simulink model "b_2x_8a_r309a"  (Simulink 6.2)
settings: Solver=ode45  StartTime=0.0  StopTime=1030.0  RelTol=1e-3
undefined symbols (not defined in the file): ant_bits, BEE2_usr, blockCountBits, blockRowBits, cmult_4bit_em
libraries: xbsIndex_r3 x3300, xps_library x102, casper_library x96
(part 8 of 22)

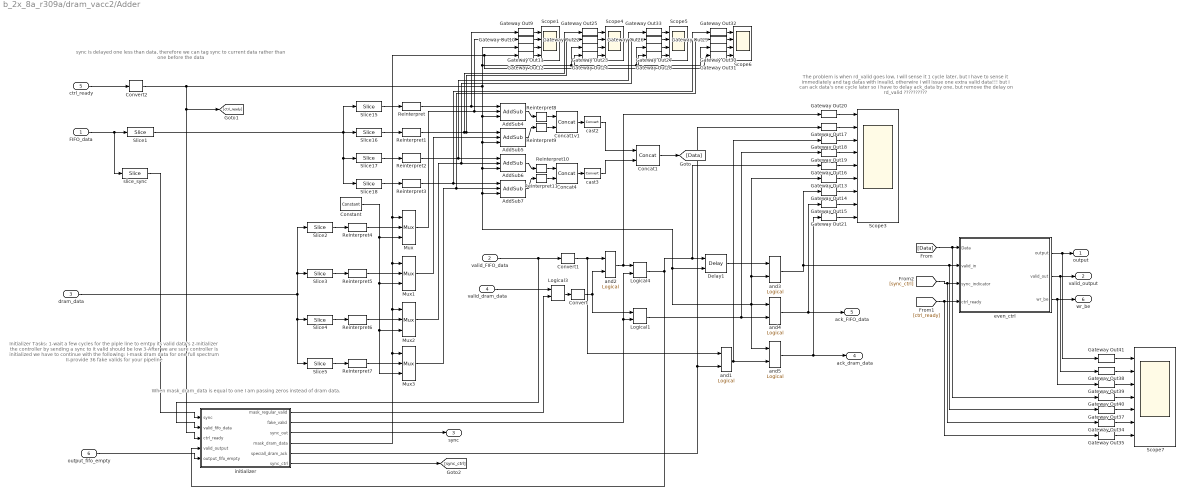
== system b_2x_8a_r309a/dram_vacc2/Adder ==
  note: When mask_dram_data is equal to one
      | I am passing zeros instead of dram data.
  note: Initializer Tasks:
      | 1-wait a few cycles for the piple line to emtpy
      | its valid data's
      | 2-Initializer the controller by sending a sync to it
      | valid should be low
      | 3-After we are sure controller is initialized we have to
      | continue with the following:
      | I-mask dram data for one full spectrum
      | II-provide 36 fake valids for your pipeline
  note: The problem is when rd_valid goes low, I will sense it 1 cycle later,
      | but I have to sense it immediately and tag datas with invalid,
      | otherwire I will issue one extra valid data!!!
      | but I can ack data's one cycle later so
      | I have to delay ack_data by one, but remove the delay on rd_valid
      | ??????????
  note: sync is delayed one less than data,
      | therefore we can tag sync to current data rather than
      | one before the data
  FIFO_data : Inport  Port=1  LatchInput=off
  valid_FIFO_data : Inport  Port=2  LatchInput=off
  dram_data : Inport  Port=3  LatchInput=off
  valid_dram_data : Inport  Port=4  LatchInput=off
  ctrl_ready : Inport  Port=5  LatchInput=off
  output_fifo_empty : Inport  Port=6  LatchInput=off
  AddSub{4..7} (4 alike) : xbsIndex_r3/AddSub  mode=Addition  precision=User Defined  arith_type="Signed  (2's comp)"  n_bits=32  bin_pt=0  quantization="Round  (unbiased: +/- Inf)"  overflow=Wrap  latency=3  explicit_period=on  period=1  use_carryin=off  use_carryout=off  en=on  dbl_ovrd=off  show_param=off  use_core=on  pipeline=on  use_rpm=on  gen_core=off
      settings: xl_area=[0, 0, 0, 0, 0, 0, 0]
  Concat1 : xbsIndex_r3/Concat  num_inputs=2  explicit_period=off  period=1  dbl_ovrd=off
  Concat1v1 : xbsIndex_r3/Concat  num_inputs=2  explicit_period=off  period=1  dbl_ovrd=off
  Concat4 : xbsIndex_r3/Concat  num_inputs=2  explicit_period=off  period=1  dbl_ovrd=off
  Constant : xbsIndex_r3/Constant  const=0  equ=P=C  arith_type="Signed  (2's comp)"  n_bits=32  bin_pt=0  opselect=C  inp2=PCIN>>17  opr=+  inp1=P  carry=CIN  iostate=0  explicit_period=on  period=1  dbl_ovrd=off
  Convert : xbsIndex_r3/Convert  arith_type=Boolean  n_bits=8  bin_pt=6  quantization=Truncate  overflow=Wrap  latency=0  explicit_period=off  period=1  dbl_ovrd=off  show_param=off  inserted_by_tool=off  pipeline=off
      settings: xl_area=[0, 0, 0, 0, 0, 0, 0]
  Convert1 : xbsIndex_r3/Convert  arith_type=Boolean  n_bits=8  bin_pt=6  quantization=Truncate  overflow=Wrap  latency=0  explicit_period=off  period=1  dbl_ovrd=off  show_param=off  inserted_by_tool=off  pipeline=off
      settings: xl_area=[0, 0, 0, 0, 0, 0, 0]
  Convert2 : xbsIndex_r3/Convert  arith_type=Boolean  n_bits=8  bin_pt=6  quantization=Truncate  overflow=Wrap  latency=0  explicit_period=off  period=1  dbl_ovrd=off  show_param=off  inserted_by_tool=off  pipeline=off
      settings: xl_area=[0, 0, 0, 0, 0, 0, 0]
  Delay1 : xbsIndex_r3/Delay  latency=3  reg_retiming=off  explicit_period=on  period=1  en=on  accept_only_valid=off  init_zero=on  dbl_ovrd=off  show_param=off
      settings: xl_area=[0, 0, 0, 0, 0, 0, 0]
  Gateway Out{9..35,37..41} (32 alike) : xbsIndex_r3/Gateway Out  output_type=Double  nbits=8  bin_pt=6  arith_type=Boolean  quantization=Truncate  overflow=Wrap  hdl_port=off  timing_constraint=None  locs_specified=off  LOCs={}  needs_fixed_name=off  show_param=off
      settings: xl_area=[0, 0, 0, 0, 0, 0, 0]
  Logical1 : xbsIndex_r3/Logical  logical_function=OR  inputs=2  precision=Full  arith_type=Unsigned  n_bits=8  bin_pt=2  align_bp=on  latency=0  explicit_period=off  period=1  en=off  dbl_ovrd=off  show_param=off
      settings: xl_area=[0, 0, 0, 0, 0, 0, 0]
  Logical3 : xbsIndex_r3/Logical  logical_function=AND  inputs=2  precision=Full  arith_type=Unsigned  n_bits=8  bin_pt=2  align_bp=on  latency=0  explicit_period=off  period=1  en=off  dbl_ovrd=off  show_param=off
      settings: xl_area=[0, 0, 0, 0, 0, 0, 0]
  Logical4 : xbsIndex_r3/Logical  logical_function=OR  inputs=2  precision=Full  arith_type=Unsigned  n_bits=8  bin_pt=2  align_bp=on  latency=0  explicit_period=off  period=1  en=off  dbl_ovrd=off  show_param=off
      settings: xl_area=[0, 0, 0, 0, 0, 0, 0]
  Mux{,1..3} (4 alike) : xbsIndex_r3/Mux  inputs=2  precision=Full  arith_type="Signed  (2's comp)"  n_bits=8  bin_pt=2  quantization=Truncate  overflow=Wrap  latency=0  explicit_period=off  period=1  en=off  dbl_ovrd=off  show_param=off  mux_type=off  use_rpm=off  gen_core=off
      settings: xl_area=[0, 0, 0, 0, 0, 0, 0]
  Reinterpret{,1..7} (8 alike) : xbsIndex_r3/Reinterpret  force_arith_type=on  arith_type="Signed  (2's comp)"  force_bin_pt=on  bin_pt=0  force_valid=on
  Reinterpret{8..11} (4 alike) : xbsIndex_r3/Reinterpret  force_arith_type=on  arith_type=Unsigned  force_bin_pt=on  bin_pt=0  force_valid=on
  Scope{1,4..6} (4 alike) : Scope  NumInputPorts=4
      Scope1 settings: YMin=0~0~0~-1  YMax=1~1750~1~1  SaveName=ScopeData30
      Scope4 settings: YMin=0~0~0~-1  YMax=1~1750~1~1  SaveName=ScopeData4
      Scope5 settings: YMin=0~0~0~-1  YMax=1~1750~1~1  SaveName=ScopeData5
      Scope6 settings: YMin=0~0~0~-1  YMax=1~1750~1~1  SaveName=ScopeData6
  Scope3 : Scope  NumInputPorts=9
      settings: YMin=0~0~0~-1~-5~-5~-5~-5~-5  YMax=1~1750~1~1~5~5~5~5~5  SaveName=ScopeData11
  Scope7 : Scope  NumInputPorts=7
      settings: YMin=0~0~0~-1~-5~-5~-5  YMax=1~1750~1~1~5~5~5  SaveName=ScopeData36
  Slice1 : xbsIndex_r3/Slice  mode=Lower Bit Location + Width  nbits=128  bit1=0  base1=MSB of Input  bit0=0  base0=LSB of Input  boolean_output=off  explicit_period=off  period=1  dbl_ovrd=off
  Slice15 : xbsIndex_r3/Slice  mode=Lower Bit Location + Width  nbits=32  bit1=96  base1=MSB of Input  bit0=96  base0=LSB of Input  boolean_output=off  explicit_period=off  period=1  dbl_ovrd=off
  Slice16 : xbsIndex_r3/Slice  mode=Lower Bit Location + Width  nbits=32  bit1=-32  base1=MSB of Input  bit0=64  base0=LSB of Input  boolean_output=off  explicit_period=off  period=1  dbl_ovrd=off
  Slice17 : xbsIndex_r3/Slice  mode=Lower Bit Location + Width  nbits=32  bit1=0  base1=MSB of Input  bit0=32  base0=LSB of Input  boolean_output=off  explicit_period=off  period=1  dbl_ovrd=off
  Slice18 : xbsIndex_r3/Slice  mode=Lower Bit Location + Width  nbits=32  bit1=0  base1=MSB of Input  bit0=0  base0=LSB of Input  boolean_output=off  explicit_period=off  period=1  dbl_ovrd=off
  Slice2 : xbsIndex_r3/Slice  mode=Lower Bit Location + Width  nbits=32  bit1=0  base1=MSB of Input  bit0=104  base0=LSB of Input  boolean_output=off  explicit_period=off  period=1  dbl_ovrd=off
  Slice3 : xbsIndex_r3/Slice  mode=Lower Bit Location + Width  nbits=32  bit1=72  base1=MSB of Input  bit0=72  base0=LSB of Input  boolean_output=off  explicit_period=off  period=1  dbl_ovrd=off
  Slice4 : xbsIndex_r3/Slice  mode=Lower Bit Location + Width  nbits=32  bit1=0  base1=MSB of Input  bit0=32  base0=LSB of Input  boolean_output=off  explicit_period=off  period=1  dbl_ovrd=off
  Slice5 : xbsIndex_r3/Slice  mode=Lower Bit Location + Width  nbits=32  bit1=0  base1=MSB of Input  bit0=0  base0=LSB of Input  boolean_output=off  explicit_period=off  period=1  dbl_ovrd=off
  and1 : xbsIndex_r3/Logical  logical_function=OR  inputs=2  precision=Full  arith_type=Unsigned  n_bits=8  bin_pt=2  align_bp=on  latency=0  explicit_period=off  period=1  en=off  dbl_ovrd=off  show_param=off
      settings: xl_area=[0, 0, 0, 0, 0, 0, 0]
  and{2..5} (4 alike) : xbsIndex_r3/Logical  logical_function=AND  inputs=2  precision=Full  arith_type=Unsigned  n_bits=8  bin_pt=2  align_bp=on  latency=0  explicit_period=off  period=1  en=off  dbl_ovrd=off  show_param=off
      settings: xl_area=[0, 0, 0, 0, 0, 0, 0]
  cast2 : xbsIndex_r3/Convert  arith_type=Unsigned  n_bits=72  bin_pt=0  quantization=Truncate  overflow=Wrap  latency=0  explicit_period=off  period=1  dbl_ovrd=off  show_param=off  inserted_by_tool=off  pipeline=off
      settings: xl_area=[0, 0, 0, 0, 0, 0, 0]
  cast3 : xbsIndex_r3/Convert  arith_type=Unsigned  n_bits=72  bin_pt=0  quantization=Truncate  overflow=Wrap  latency=0  explicit_period=off  period=1  dbl_ovrd=off  show_param=off  inserted_by_tool=off  pipeline=off
      settings: xl_area=[0, 0, 0, 0, 0, 0, 0]
  even_ctrl : Subsystem
  initializer : Subsystem
  slice_sync : xbsIndex_r3/Slice  mode=Upper Bit Location + Width  nbits=1  bit1=0  base1=MSB of Input  bit0=0  base0=LSB of Input  boolean_output=on  explicit_period=off  period=1  dbl_ovrd=off
  output : Outport
  valid_output : Outport  Port=2
  sync : Outport  Port=3
  ack_dram_data : Outport  Port=4
  ack_FIFO_data : Outport  Port=5
  wr_be : Outport  Port=6
  wires:
  Gateway Out31/1 -> Scope6/4
  Gateway Out30/1 -> Scope6/3
  Gateway Out29/1 -> Scope6/2
  Gateway Out32/1 -> Scope6/1
  Gateway Out28/1 -> Scope5/4
  Gateway Out27/1 -> Scope5/3
  Gateway Out26/1 -> Scope5/2
  Gateway Out33/1 -> Scope5/1
  Gateway Out24/1 -> Scope4/4
  Gateway Out23/1 -> Scope4/3
  Gateway Out22/1 -> Scope4/2
  Gateway Out25/1 -> Scope4/1
  Reinterpret11/1 -> Concat4/2
  Reinterpret10/1 -> Concat4/1
  Reinterpret9/1 -> Concat1v1/2
  Reinterpret8/1 -> Concat1v1/1
  Reinterpret7/1 -> Mux3/2
  Reinterpret6/1 -> Mux2/2
  Reinterpret5/1 -> Mux1/2
  Reinterpret4/1 -> Mux/2
  Reinterpret3/1 -> Gateway Out32/1, AddSub7/1
  Reinterpret2/1 -> Gateway Out33/1, AddSub6/1
  Reinterpret1/1 -> Gateway Out22/1, AddSub5/1, Gateway Out25/1
  Reinterpret/1 -> Gateway Out9/1, AddSub4/1
  Logical1/1 -> Gateway Out19/1, and4/2
  Gateway Out21/1 -> Scope3/9
  Gateway Out15/1 -> Scope3/8
  Gateway Out14/1 -> Scope3/7
  Gateway Out13/1 -> Scope3/6
  Gateway Out16/1 -> Scope3/5
  Gateway Out18/1 -> Scope3/3
  Gateway Out19/1 -> Scope3/4
  Gateway Out17/1 -> Scope3/2
  Gateway Out20/1 -> Scope3/1
  and1/1 -> Gateway Out18/1, and5/2
  and5/1 -> Gateway Out21/1, ack_dram_data/1
  Logical4/1 -> Gateway Out16/1, Delay1/1, initializer/4(valid_output)
  Gateway Out12/1 -> Scope1/4
  Gateway Out11/1 -> Scope1/3
  Gateway Out10/1 -> Scope1/2
  Gateway Out9/1 -> Scope1/1
  initializer/5(speciall_dram_ack) -> Gateway Out17/1, and1/2
  output_fifo_empty/1 -> initializer/5(output_fifo_empty)
  Constant/1 -> Mux2/3, Mux3/3, Mux1/3, Mux/3
  initializer/4(mask_dram_data) -> Mux3/1, Mux2/1, Gateway Out31/1, Gateway Out28/1, Gateway Out24/1, Gateway Out12/1, Mux/1, Mux1/1
  Slice2/1 -> Reinterpret4/1
  Slice3/1 -> Reinterpret5/1
  Slice4/1 -> Reinterpret6/1
  Slice5/1 -> Reinterpret7/1
  initializer/3(sync_out) -> sync/1
  and2/1 -> Gateway Out20/1, Logical4/1
  and4/1 -> Gateway Out15/1, ack_FIFO_data/1
  Delay1/1 -> and3/1
  initializer/2(fake_valid) -> Logical1/2, Logical4/2
  Logical3/1 -> Convert/1
  initializer/1(mask_regular_valid) -> Logical3/2
  valid_dram_data/1 -> Logical3/1
  and3/1 -> Gateway Out14/1, even_ctrl/2(valid_in), Gateway Out37/1
  Convert2/1 -> Gateway Out30/1, Gateway Out27/1, Gateway Out23/1, Gateway Out11/1, AddSub4/3, AddSub5/3, Delay1/2, Gateway Out13/1, and3/2, and5/1, and4/1, AddSub7/3, AddSub6/3, [ctrl_ready], initializer/3(ctrl_ready)
  Convert1/1 -> and1/1, and2/1
  Convert/1 -> Logical1/1, and2/2
  slice_sync/1 -> initializer/1(sync)
  Slice1/1 -> Slice18/1, Slice17/1, Slice16/1, Slice15/1
  dram_data/1 -> Slice4/1, Slice5/1, Slice3/1, Slice2/1
  valid_FIFO_data/1 -> Convert1/1, initializer/2(valid_fifo_data)
  ctrl_ready/1 -> Convert2/1
  FIFO_data/1 -> slice_sync/1, Slice1/1
  cast3/1 -> Concat1/2
  Concat4/1 -> cast3/1
  cast2/1 -> Concat1/1
  Concat1v1/1 -> cast2/1
  AddSub7/1 -> Reinterpret11/1
  AddSub6/1 -> Reinterpret10/1
  AddSub5/1 -> Reinterpret9/1
  AddSub4/1 -> Reinterpret8/1
  Mux3/1 -> Gateway Out29/1, AddSub7/2
  Mux2/1 -> Gateway Out26/1, AddSub6/2
  Mux1/1 -> AddSub5/2
  Mux/1 -> Gateway Out10/1, AddSub4/2
  Slice18/1 -> Reinterpret3/1
  Slice17/1 -> Reinterpret2/1
  Slice16/1 -> Reinterpret1/1
  Slice15/1 -> Reinterpret/1
  even_ctrl/1(output) -> output/1, Gateway Out41/1
  even_ctrl/2(valid_out) -> valid_output/1, Gateway Out38/1
  Concat1/1 -> [Data]
  [Data] -> even_ctrl/1(Data), Gateway Out40/1
  [ctrl_ready] -> even_ctrl/4(ctrl_ready), Gateway Out35/1
  even_ctrl/3(wr_be) -> wr_be/1, Gateway Out39/1
  initializer/6(sync_ctrl) -> [sync_ctrl]
  [sync_ctrl] -> even_ctrl/3(sync_indicator), Gateway Out34/1
  Gateway Out35/1 -> Scope7/7
  Gateway Out34/1 -> Scope7/6
  Gateway Out37/1 -> Scope7/5
  Gateway Out39/1 -> Scope7/3
  Gateway Out40/1 -> Scope7/4
  Gateway Out38/1 -> Scope7/2
  Gateway Out41/1 -> Scope7/1

== system b_2x_8a_r309a/dram_vacc2/RB_reg ==
  note: HIgh bit of tag means its a read back
      | and low bit means its a valid read back
      | This module has to ack dram for all
      | rd backs (even invalid ones)
      | but it neads to only capture valid
      | read backs.
  note: if this is high it means data is a RB data
  dram_data : Inport  Port=1  LatchInput=off
  rd_tag : Inport  Port=2  LatchInput=off
  rd_valid : Inport  Port=3  LatchInput=off
  dram_rd_ack : Inport  Port=4  LatchInput=off
  ack_RB : Inport  Port=5  LatchInput=off
  RB_active : Inport  Port=6  LatchInput=off
  Concat : xbsIndex_r3/Concat  num_inputs=2  explicit_period=off  period=1  dbl_ovrd=off
  Convert{1..2,4..5} (4 alike) : xbsIndex_r3/Convert  arith_type=Boolean  n_bits=31  bin_pt=0  quantization=Truncate  overflow=Wrap  latency=0  explicit_period=off  period=1  dbl_ovrd=off  show_param=off  inserted_by_tool=off  pipeline=off
      settings: xl_area=[0, 0, 0, 0, 0, 0, 0]
  Delay : xbsIndex_r3/Delay  latency=1  reg_retiming=on  explicit_period=off  period=1  en=off  accept_only_valid=off  init_zero=on  dbl_ovrd=off  show_param=off
      settings: xl_area=[0, 0, 0, 0, 0, 0, 0]
  Inverter2 : xbsIndex_r3/Inverter  latency=0  explicit_period=off  period=1  en=off  dbl_ovrd=off  show_param=off
      settings: xl_area=[0, 0, 0, 0, 0, 0, 0]
  Logical1 : xbsIndex_r3/Logical  logical_function=AND  inputs=2  precision=Full  arith_type=Unsigned  n_bits=8  bin_pt=2  align_bp=on  latency=0  explicit_period=on  period=1  en=off  dbl_ovrd=off  show_param=off
      settings: xl_area=[0, 0, 0, 0, 0, 0, 0]
  Logical2 : xbsIndex_r3/Logical  logical_function=AND  inputs=4  precision=Full  arith_type=Unsigned  n_bits=8  bin_pt=2  align_bp=on  latency=0  explicit_period=on  period=1  en=off  dbl_ovrd=off  show_param=off
      settings: xl_area=[0, 0, 0, 0, 0, 0, 0]
  Logical3 : xbsIndex_r3/Logical  logical_function=AND  inputs=2  precision=Full  arith_type=Unsigned  n_bits=8  bin_pt=2  align_bp=on  latency=0  explicit_period=on  period=1  en=off  dbl_ovrd=off  show_param=off
      settings: xl_area=[0, 0, 0, 0, 0, 0, 0]
  Logical4 : xbsIndex_r3/Logical  logical_function=OR  inputs=2  precision=Full  arith_type=Unsigned  n_bits=8  bin_pt=2  align_bp=on  latency=0  explicit_period=on  period=1  en=off  dbl_ovrd=off  show_param=off
      settings: xl_area=[0, 0, 0, 0, 0, 0, 0]
  Register : xbsIndex_r3/Register  init=0  reg_only_valid=off  explicit_period=off  period=1  rst=on  en=on  out_en=off  dbl_ovrd=off  show_param=off
      settings: xl_area=[0, 0, 0, 0, 0, 0, 0]
  Reinterpret : xbsIndex_r3/Reinterpret  force_arith_type=on  arith_type=Unsigned  force_bin_pt=on  bin_pt=0  force_valid=on
  Slice : xbsIndex_r3/Slice  mode=Lower Bit Location + Width  nbits=64  bit1=0  base1=MSB of Input  bit0=72  base0=LSB of Input  boolean_output=off  explicit_period=off  period=1  dbl_ovrd=off
  Slice1 : xbsIndex_r3/Slice  mode=Lower Bit Location + Width  nbits=64  bit1=0  base1=MSB of Input  bit0=0  base0=LSB of Input  boolean_output=off  explicit_period=off  period=1  dbl_ovrd=off
  Slice2 : xbsIndex_r3/Slice  mode=Upper Bit Location + Width  nbits=1  bit1=0  base1=MSB of Input  bit0=74  base0=LSB of Input  boolean_output=on  explicit_period=off  period=1  dbl_ovrd=off
  Slice3 : xbsIndex_r3/Slice  mode=Lower Bit Location + Width  nbits=1  bit1=0  base1=MSB of Input  bit0=0  base0=LSB of Input  boolean_output=on  explicit_period=off  period=1  dbl_ovrd=off
  Trickle_FWFT : Subsystem  mask{depth=16}
      mask init:
      | cursys = gcb ; 
      | set_param([cursys, '/FIFO'], 'depth', depth);
      mask StyleString: popup(16|32|64|128|256|512|1K|2K|4K|8K|16K|32K|64K)
  posedge : Subsystem
  dout : Outport
  valid : Outport  Port=2
  ack_dram : Outport  Port=3
  en_addr_gen : Outport  Port=4
  wires:
  Reinterpret/1 -> Inverter2/1
  Convert2/1 -> Logical3/1
  Slice3/1 -> Logical2/4
  Slice2/1 -> Logical1/1
  Convert4/1 -> Logical1/2
  Logical4/1 -> Register/2
  Register/1 -> Logical3/2
  Logical3/1 -> Logical4/2, en_addr_gen/1
  Inverter2/1 -> Convert2/1
  Trickle_FWFT/4(%full) -> Reinterpret/1
  Trickle_FWFT/2(valid) -> valid/1
  Trickle_FWFT/1(data_out) -> dout/1
  posedge/1(out) -> Logical4/1, Trickle_FWFT/4(reset)
  Concat/1 -> Trickle_FWFT/1(din)
  ack_RB/1 -> Trickle_FWFT/3(ack)
  Convert1/1 -> Logical2/3, posedge/1(in)
  dram_data/1 -> Slice1/1, Slice/1
  Slice1/1 -> Concat/2
  Slice/1 -> Concat/1
  Convert5/1 -> Logical2/2
  RB_active/1 -> Convert1/1
  Logical2/1 -> Register/3, Register/1, Trickle_FWFT/2(we)
  dram_rd_ack/1 -> Convert5/1
  Logical1/1 -> Logical2/1, Delay/1
  Delay/1 -> ack_dram/1
  rd_valid/1 -> Convert4/1
  rd_tag/1 -> Slice3/1, Slice2/1

== system b_2x_8a_r309a/dram_vacc2/Trickle_FWFT ==
  note: We needed a FIFO which brings the valid data automatically to the output.
      | The regular XILINX Fifos are not FWFT (First Word Fall Through).
      | We tried to make one but it was really hard to make one agreeing with the exact specs.
      | This module which we have named it Trickle_FWFT Fifo works very similiarly with minor
      | differences which servers our purpose here in the DRAM VACC module.
  note: The real depth of this module is depth+1.
      | The valid signal will go high with one cycle delay.
  din : Inport  Port=1  LatchInput=off
  we : Inport  Port=2  LatchInput=off
  ack : Inport  Port=3  LatchInput=off
  reset : Inport  Port=4  LatchInput=off
  Convert : xbsIndex_r3/Convert  Orientation=left  arith_type=Boolean  n_bits=8  bin_pt=6  quantization=Truncate  overflow=Wrap  latency=0  explicit_period=on  period=1  dbl_ovrd=off  show_param=off  inserted_by_tool=off  pipeline=off
      settings: xl_area=[0, 0, 0, 0, 0, 0, 0]
  Convert1 : xbsIndex_r3/Convert  arith_type=Boolean  n_bits=8  bin_pt=6  quantization=Truncate  overflow=Wrap  latency=0  explicit_period=off  period=1  dbl_ovrd=off  show_param=off  inserted_by_tool=off  pipeline=off
      settings: xl_area=[0, 0, 0, 0, 0, 0, 0]
  Convert2 : xbsIndex_r3/Convert  arith_type=Boolean  n_bits=8  bin_pt=6  quantization=Truncate  overflow=Wrap  latency=0  explicit_period=off  period=1  dbl_ovrd=off  show_param=off  inserted_by_tool=off  pipeline=off
      settings: xl_area=[0, 0, 0, 0, 0, 0, 0]
  FIFO : xbsIndex_r3/FIFO  depth=512  percent_nbits=1  store_only_valid=on  init_zero=on  explicit_period=on  period=1  rst=on  en=off  use_almost_empty=off  almost_empty_offset=6  use_almost_full=off  almost_full_offset=6  dbl_ovrd=off  show_param=off  mem_type=Block RAM  gen_core=off
      settings: xl_area=[0, 0, 0, 0, 0, 0, 0]
  Inverter3 : xbsIndex_r3/Inverter  latency=0  explicit_period=off  period=1  en=off  dbl_ovrd=off  show_param=off
      settings: xl_area=[0, 0, 0, 0, 0, 0, 0]
  Logical2 : xbsIndex_r3/Logical  logical_function=OR  inputs=2  precision=Full  arith_type=Unsigned  n_bits=8  bin_pt=2  align_bp=on  latency=0  explicit_period=on  period=1  en=off  dbl_ovrd=off  show_param=off
      settings: xl_area=[0, 0, 0, 0, 0, 0, 0]
  not_valid : xbsIndex_r3/Register  init=1  reg_only_valid=off  explicit_period=on  period=1  rst=on  en=on  out_en=off  dbl_ovrd=off  show_param=off
      settings: xl_area=[0, 0, 0, 0, 0, 0, 0]
  data_out : Outport
  valid : Outport  Port=2
  full : Outport  Port=3
  %full : Outport  Port=4
  wires:
  din/1 -> FIFO/1
  we/1 -> FIFO/2
  FIFO/2 -> not_valid/1
  ack/1 -> Convert2/1
  FIFO/1 -> data_out/1
  FIFO/4 -> full/1
  Inverter3/1 -> valid/1
  reset/1 -> FIFO/4, not_valid/2
  Logical2/1 -> FIFO/3, not_valid/3
  not_valid/1 -> Convert1/1
  Convert/1 -> Logical2/1
  FIFO/3 -> %full/1
  Convert1/1 -> Inverter3/1, Convert/1
  Convert2/1 -> Logical2/2

== system b_2x_8a_r309a/dram_vacc2/ctrl_unit ==
  valid_data : Inport  Port=1  LatchInput=off
  sync : Inport  Port=2  LatchInput=off
  en_RB_addr : Inport  Port=3  LatchInput=off
  Concat1 : xbsIndex_r3/Concat  num_inputs=3  explicit_period=off  period=1  dbl_ovrd=off
  Convert2 : xbsIndex_r3/Convert  arith_type=Unsigned  n_bits=30  bin_pt=0  quantization=Truncate  overflow=Wrap  latency=0  explicit_period=off  period=1  dbl_ovrd=off  show_param=off  inserted_by_tool=off  pipeline=off
      settings: xl_area=[0, 0, 0, 0, 0, 0, 0]
  Delay1 : xbsIndex_r3/Delay  latency=2  reg_retiming=off  explicit_period=on  period=1  en=off  accept_only_valid=off  init_zero=on  dbl_ovrd=off  show_param=off
      settings: xl_area=[0, 0, 0, 0, 0, 0, 0]
  Delay2 : xbsIndex_r3/Delay  latency=1  reg_retiming=off  explicit_period=on  period=1  en=off  accept_only_valid=off  init_zero=on  dbl_ovrd=off  show_param=off
      settings: xl_area=[0, 0, 0, 0, 0, 0, 0]
  Mux : xbsIndex_r3/Mux  inputs=2  precision=Full  arith_type="Signed  (2's comp)"  n_bits=8  bin_pt=2  quantization=Truncate  overflow=Wrap  latency=0  explicit_period=off  period=1  en=off  dbl_ovrd=off  show_param=off  mux_type=off  use_rpm=off  gen_core=off
      settings: xl_area=[0, 0, 0, 0, 0, 0, 0]
  Mux2 : xbsIndex_r3/Mux  inputs=2  precision=Full  arith_type="Signed  (2's comp)"  n_bits=8  bin_pt=2  quantization=Truncate  overflow=Wrap  latency=0  explicit_period=off  period=1  en=off  dbl_ovrd=off  show_param=off  mux_type=off  use_rpm=off  gen_core=off
      settings: xl_area=[0, 0, 0, 0, 0, 0, 0]
  RB_active_or_finish : Subsystem
  address_gen_vacc_DRAM : Subsystem  mask{acc_length=acc_length, valid_length=burst_length}
      mask prompts: acc_length "Accumulation length?"; valid_length "Valid period length?"
      mask init:
      | address_gen_vacc_v2_mask;
  cmd_gen : Subsystem
  latch_rb_enable : Subsystem
  negedge : Subsystem  Orientation=down
  readback_address_dram_vacc : Subsystem  mask{acc_length=acc_length, valid_length=valid_length}
      mask prompts: acc_length "Accumulation length?"; valid_length "Valid period length?"
      mask init:
      | readback_address_dram_vacc_mask;
  address : Outport
  cmd_tag : Outport  Port=2
  RB_active : Outport  Port=3
  RWn : Outport  Port=4
  cmd_valid : Outport  Port=5
  ready : Outport  Port=6
  wires:
  latch_rb_enable/2(cmd_tag) -> Concat1/3
  Delay1/1 -> latch_rb_enable/1(sync), readback_address_dram_vacc/1(sync)  "v"
  negedge/1(out) -> latch_rb_enable/3(negedge)
  latch_rb_enable/1(inc_addr_en) -> RB_active_or_finish/1(enable_rb_addr), readback_address_dram_vacc/2(en)
  readback_address_dram_vacc/1(readback_addr) -> Mux2/3
  valid_data/1 -> cmd_gen/1(valid_data)
  cmd_gen/6(rb_addr_en) -> negedge/1(in), Concat1/1, Mux2/1
  cmd_gen/5(ready) -> ready/1
  cmd_gen/4(cmd_valid) -> cmd_valid/1
  cmd_gen/3(RWn) -> Mux/1, RWn/1
  RB_active_or_finish/1(rb_active) -> RB_active/1
  Mux2/1 -> address/1, Convert2/1
  en_RB_addr/1 -> latch_rb_enable/2(rb_addr_enable)
  Delay2/1 -> address_gen_vacc_DRAM/1(sync)
  Concat1/1 -> cmd_tag/1
  Convert2/1 -> Concat1/2
  cmd_gen/2(wr_addr_en) -> address_gen_vacc_DRAM/3(write_en)
  cmd_gen/1(re_addr_en) -> address_gen_vacc_DRAM/2(read_en)
  Mux/1 -> Mux2/2
  address_gen_vacc_DRAM/2(read_addr) -> Mux/3
  address_gen_vacc_DRAM/1(write_addr) -> Mux/2
  sync/1 -> Delay2/1, RB_active_or_finish/2(sync), Delay1/1, cmd_gen/2(sync)

== system b_2x_8a_r309a/dram_vacc2/dram1 ==
  rst : Inport  Port=1  LatchInput=off
  address : Inport  Port=2  LatchInput=off
  data_in : Inport  Port=3  LatchInput=off
  wr_be : Inport  Port=4  LatchInput=off
  RWn : Inport  Port=5  LatchInput=off
  cmd_tag : Inport  Port=6  LatchInput=off
  cmd_valid : Inport  Port=7  LatchInput=off
  rd_ack : Inport  Port=8  LatchInput=off
  Constant : Constant  Value=0
  Simulation Multiplexer{,1..3} (4 alike) : xbsIndex_r3/Simulation Multiplexer  sim_sel=2  hw_sel=1
  Terminator{,1..7} (8 alike) : Terminator
  b_2x_8a_r309a_dram_vacc2_dram1_Mem_Cmd_Ack : xbsIndex_r3/Gateway In  arith_type=Unsigned  n_bits=1  bin_pt=0  quantization=Truncate  overflow=Wrap  period=sample_period  timing_constraint=None  locs_specified=off  LOCs={}  needs_fixed_name=off  dbl_ovrd=off  show_param=off
      settings: xl_area=[0, 0, 0, 0, 0, 0, 0]
  b_2x_8a_r309a_dram_vacc2_dram1_Mem_Cmd_Address : xbsIndex_r3/Gateway Out  output_type=Double  nbits=8  bin_pt=6  arith_type=Boolean  quantization=Truncate  overflow=Wrap  hdl_port=on  timing_constraint=None  locs_specified=off  LOCs={}  needs_fixed_name=off  show_param=off
      settings: xl_area=[0, 0, 0, 0, 0, 0, 0]
  b_2x_8a_r309a_dram_vacc2_dram1_Mem_Cmd_RNW : xbsIndex_r3/Gateway Out  output_type=Double  nbits=8  bin_pt=6  arith_type=Boolean  quantization=Truncate  overflow=Wrap  hdl_port=on  timing_constraint=None  locs_specified=off  LOCs={}  needs_fixed_name=off  show_param=off
      settings: xl_area=[0, 0, 0, 0, 0, 0, 0]
  b_2x_8a_r309a_dram_vacc2_dram1_Mem_Cmd_Tag : xbsIndex_r3/Gateway Out  output_type=Double  nbits=8  bin_pt=6  arith_type=Boolean  quantization=Truncate  overflow=Wrap  hdl_port=on  timing_constraint=None  locs_specified=off  LOCs={}  needs_fixed_name=off  show_param=off
      settings: xl_area=[0, 0, 0, 0, 0, 0, 0]
  b_2x_8a_r309a_dram_vacc2_dram1_Mem_Cmd_Valid : xbsIndex_r3/Gateway Out  output_type=Double  nbits=8  bin_pt=6  arith_type=Boolean  quantization=Truncate  overflow=Wrap  hdl_port=on  timing_constraint=None  locs_specified=off  LOCs={}  needs_fixed_name=off  show_param=off
      settings: xl_area=[0, 0, 0, 0, 0, 0, 0]
  b_2x_8a_r309a_dram_vacc2_dram1_Mem_Rd_Ack : xbsIndex_r3/Gateway Out  output_type=Double  nbits=8  bin_pt=6  arith_type=Boolean  quantization=Truncate  overflow=Wrap  hdl_port=on  timing_constraint=None  locs_specified=off  LOCs={}  needs_fixed_name=off  show_param=off
      settings: xl_area=[0, 0, 0, 0, 0, 0, 0]
  b_2x_8a_r309a_dram_vacc2_dram1_Mem_Rd_Dout : xbsIndex_r3/Gateway In  arith_type=Unsigned  n_bits=144  bin_pt=0  quantization=Truncate  overflow=Wrap  period=sample_period  timing_constraint=None  locs_specified=off  LOCs={}  needs_fixed_name=off  dbl_ovrd=off  show_param=off
      settings: xl_area=[0, 0, 0, 0, 0, 0, 0]
  b_2x_8a_r309a_dram_vacc2_dram1_Mem_Rd_Tag : xbsIndex_r3/Gateway In  arith_type=Unsigned  n_bits=32  bin_pt=0  quantization=Truncate  overflow=Wrap  period=sample_period  timing_constraint=None  locs_specified=off  LOCs={}  needs_fixed_name=off  dbl_ovrd=off  show_param=off
      settings: xl_area=[0, 0, 0, 0, 0, 0, 0]
  b_2x_8a_r309a_dram_vacc2_dram1_Mem_Rd_Valid : xbsIndex_r3/Gateway In  arith_type=Unsigned  n_bits=1  bin_pt=0  quantization=Truncate  overflow=Wrap  period=sample_period  timing_constraint=None  locs_specified=off  LOCs={}  needs_fixed_name=off  dbl_ovrd=off  show_param=off
      settings: xl_area=[0, 0, 0, 0, 0, 0, 0]
  b_2x_8a_r309a_dram_vacc2_dram1_Mem_Rst : xbsIndex_r3/Gateway Out  output_type=Double  nbits=8  bin_pt=6  arith_type=Boolean  quantization=Truncate  overflow=Wrap  hdl_port=on  timing_constraint=None  locs_specified=off  LOCs={}  needs_fixed_name=off  show_param=off
      settings: xl_area=[0, 0, 0, 0, 0, 0, 0]
  b_2x_8a_r309a_dram_vacc2_dram1_Mem_Wr_BE : xbsIndex_r3/Gateway Out  output_type=Double  nbits=8  bin_pt=6  arith_type=Boolean  quantization=Truncate  overflow=Wrap  hdl_port=on  timing_constraint=None  locs_specified=off  LOCs={}  needs_fixed_name=off  show_param=off
      settings: xl_area=[0, 0, 0, 0, 0, 0, 0]
  b_2x_8a_r309a_dram_vacc2_dram1_Mem_Wr_Din : xbsIndex_r3/Gateway Out  output_type=Double  nbits=8  bin_pt=6  arith_type=Boolean  quantization=Truncate  overflow=Wrap  hdl_port=on  timing_constraint=None  locs_specified=off  LOCs={}  needs_fixed_name=off  show_param=off
      settings: xl_area=[0, 0, 0, 0, 0, 0, 0]
  convert_address : xbsIndex_r3/Convert  arith_type=Unsigned  n_bits=32  bin_pt=0  quantization=Truncate  overflow=Wrap  latency=0  explicit_period=off  period=sample_period  dbl_ovrd=off  show_param=off  inserted_by_tool=off  pipeline=off
      settings: xl_area=[0, 0, 0, 0, 0, 0, 0]
  convert_cmd_tag : xbsIndex_r3/Convert  arith_type=Unsigned  n_bits=32  bin_pt=0  quantization=Truncate  overflow=Wrap  latency=0  explicit_period=off  period=1  dbl_ovrd=off  show_param=off  inserted_by_tool=off  pipeline=off
      settings: xl_area=[0, 0, 0, 0, 0, 0, 0]
  convert_cmd_valid : xbsIndex_r3/Convert  arith_type=Unsigned  n_bits=1  bin_pt=0  quantization=Truncate  overflow=Wrap  latency=0  explicit_period=off  period=1  dbl_ovrd=off  show_param=off  inserted_by_tool=off  pipeline=off
      settings: xl_area=[0, 0, 0, 0, 0, 0, 0]
  convert_data_in : xbsIndex_r3/Convert  arith_type=Unsigned  n_bits=144  bin_pt=0  quantization=Truncate  overflow=Wrap  latency=0  explicit_period=off  period=sample_period  dbl_ovrd=off  show_param=off  inserted_by_tool=off  pipeline=off
      settings: xl_area=[0, 0, 0, 0, 0, 0, 0]
  convert_rd_ack : xbsIndex_r3/Convert  arith_type=Unsigned  n_bits=1  bin_pt=0  quantization=Truncate  overflow=Wrap  latency=0  explicit_period=off  period=1  dbl_ovrd=off  show_param=off  inserted_by_tool=off  pipeline=off
      settings: xl_area=[0, 0, 0, 0, 0, 0, 0]
  convert_rst : xbsIndex_r3/Convert  arith_type=Unsigned  n_bits=1  bin_pt=0  quantization=Truncate  overflow=Wrap  latency=0  explicit_period=off  period=sample_period  dbl_ovrd=off  show_param=off  inserted_by_tool=off  pipeline=off
      settings: xl_area=[0, 0, 0, 0, 0, 0, 0]
  convert_rwn : xbsIndex_r3/Convert  arith_type=Unsigned  n_bits=1  bin_pt=0  quantization=Truncate  overflow=Wrap  latency=0  explicit_period=off  period=1  dbl_ovrd=off  show_param=off  inserted_by_tool=off  pipeline=off
      settings: xl_area=[0, 0, 0, 0, 0, 0, 0]
  convert_wr_be : xbsIndex_r3/Convert  arith_type=Unsigned  n_bits=18  bin_pt=0  quantization=Truncate  overflow=Wrap  latency=0  explicit_period=off  period=1  dbl_ovrd=off  show_param=off  inserted_by_tool=off  pipeline=off
      settings: xl_area=[0, 0, 0, 0, 0, 0, 0]
  force_data_in : xbsIndex_r3/Reinterpret  force_arith_type=on  arith_type=Unsigned  force_bin_pt=on  bin_pt=0  force_valid=on
  force_rd_dout : xbsIndex_r3/Reinterpret  force_arith_type=on  arith_type=Unsigned  force_bin_pt=on  bin_pt=0  force_valid=on
  sim_wrapper : Subsystem
  cmd_ack : Outport
  data_out : Outport  Port=2
  rd_tag : Outport  Port=3
  rd_valid : Outport  Port=4
  wires:
  force_rd_dout/1 -> data_out/1
  force_data_in/1 -> b_2x_8a_r309a_dram_vacc2_dram1_Mem_Wr_Din/1, sim_wrapper/3(data_in)
  convert_rd_ack/1 -> b_2x_8a_r309a_dram_vacc2_dram1_Mem_Rd_Ack/1, sim_wrapper/8(rd_ack)
  convert_cmd_valid/1 -> b_2x_8a_r309a_dram_vacc2_dram1_Mem_Cmd_Valid/1, sim_wrapper/7(cmd_valid)
  convert_cmd_tag/1 -> b_2x_8a_r309a_dram_vacc2_dram1_Mem_Cmd_Tag/1, sim_wrapper/6(cmd_tag)
  convert_rwn/1 -> b_2x_8a_r309a_dram_vacc2_dram1_Mem_Cmd_RNW/1, sim_wrapper/5(RWn)
  convert_wr_be/1 -> b_2x_8a_r309a_dram_vacc2_dram1_Mem_Wr_BE/1, sim_wrapper/4(wr_be)
  convert_data_in/1 -> force_data_in/1
  convert_address/1 -> b_2x_8a_r309a_dram_vacc2_dram1_Mem_Cmd_Address/1, sim_wrapper/2(address)
  convert_rst/1 -> b_2x_8a_r309a_dram_vacc2_dram1_Mem_Rst/1, sim_wrapper/1(rst)
  rd_ack/1 -> convert_rd_ack/1
  cmd_valid/1 -> convert_cmd_valid/1
  cmd_tag/1 -> convert_cmd_tag/1
  RWn/1 -> convert_rwn/1
  data_in/1 -> convert_data_in/1
  rst/1 -> convert_rst/1
  address/1 -> convert_address/1
  wr_be/1 -> convert_wr_be/1
  b_2x_8a_r309a_dram_vacc2_dram1_Mem_Rst/1 -> Terminator/1
  b_2x_8a_r309a_dram_vacc2_dram1_Mem_Cmd_Address/1 -> Terminator1/1
  b_2x_8a_r309a_dram_vacc2_dram1_Mem_Wr_Din/1 -> Terminator2/1
  b_2x_8a_r309a_dram_vacc2_dram1_Mem_Wr_BE/1 -> Terminator3/1
  b_2x_8a_r309a_dram_vacc2_dram1_Mem_Cmd_RNW/1 -> Terminator4/1
  b_2x_8a_r309a_dram_vacc2_dram1_Mem_Cmd_Tag/1 -> Terminator5/1
  b_2x_8a_r309a_dram_vacc2_dram1_Mem_Cmd_Valid/1 -> Terminator6/1
  b_2x_8a_r309a_dram_vacc2_dram1_Mem_Rd_Ack/1 -> Terminator7/1
  Constant/1 -> b_2x_8a_r309a_dram_vacc2_dram1_Mem_Cmd_Ack/1, b_2x_8a_r309a_dram_vacc2_dram1_Mem_Rd_Dout/1, b_2x_8a_r309a_dram_vacc2_dram1_Mem_Rd_Tag/1, b_2x_8a_r309a_dram_vacc2_dram1_Mem_Rd_Valid/1
  b_2x_8a_r309a_dram_vacc2_dram1_Mem_Cmd_Ack/1 -> Simulation Multiplexer/1
  Simulation Multiplexer/1 -> cmd_ack/1
  b_2x_8a_r309a_dram_vacc2_dram1_Mem_Rd_Dout/1 -> Simulation Multiplexer1/1
  Simulation Multiplexer1/1 -> force_rd_dout/1
  Simulation Multiplexer2/1 -> rd_tag/1
  Simulation Multiplexer3/1 -> rd_valid/1
  b_2x_8a_r309a_dram_vacc2_dram1_Mem_Rd_Tag/1 -> Simulation Multiplexer2/1
  b_2x_8a_r309a_dram_vacc2_dram1_Mem_Rd_Valid/1 -> Simulation Multiplexer3/1
  sim_wrapper/1(cmd_ack) -> Simulation Multiplexer/2
  sim_wrapper/2(data_out) -> Simulation Multiplexer1/2
  sim_wrapper/3(rd_tag) -> Simulation Multiplexer2/2
  sim_wrapper/4(rd_valid) -> Simulation Multiplexer3/2

== system b_2x_8a_r309a/dram_vacc2/fifo_empty_check ==
  cmd_valid : Inport  Port=1  LatchInput=off
  tag_in : Inport  Port=2  LatchInput=off
  RWn : Inport  Port=3  LatchInput=off
  dram_data_tag : Inport  Port=4  LatchInput=off
  rd_ack : Inport  Port=5  LatchInput=off
  rd_valid : Inport  Port=6  LatchInput=off
  Convert : xbsIndex_r3/Convert  arith_type=Boolean  n_bits=8  bin_pt=6  quantization=Truncate  overflow=Wrap  latency=0  explicit_period=off  period=1  dbl_ovrd=off  show_param=off  inserted_by_tool=off  pipeline=off
      settings: xl_area=[0, 0, 0, 0, 0, 0, 0]
  Counter : xbsIndex_r3/Counter  cnt_type=Free Running  n_bits=1  bin_pt=0  arith_type=Unsigned  start_count=0  cnt_to=Inf  cnt_by_val=1  operation=Up  explicit_period=off  period=1  load_pin=off  rst=off  en=on  dbl_ovrd=off  show_param=off  use_rpm=on  gen_core=off
      settings: xl_area=[0, 0, 0, 0, 0, 0, 0]
  Delay1 : xbsIndex_r3/Delay  latency=1  reg_retiming=off  explicit_period=off  period=1  en=off  accept_only_valid=off  init_zero=on  dbl_ovrd=off  show_param=off
      settings: xl_area=[0, 0, 0, 0, 0, 0, 0]
  Delay2 : xbsIndex_r3/Delay  latency=1  reg_retiming=off  explicit_period=off  period=1  en=off  accept_only_valid=off  init_zero=on  dbl_ovrd=off  show_param=off
      settings: xl_area=[0, 0, 0, 0, 0, 0, 0]
  Gateway Out{1..2,32..38} (9 alike) : xbsIndex_r3/Gateway Out  output_type=Double  nbits=8  bin_pt=6  arith_type=Boolean  quantization=Truncate  overflow=Wrap  hdl_port=off  timing_constraint=None  locs_specified=off  LOCs={}  needs_fixed_name=off  show_param=off
      settings: xl_area=[0, 0, 0, 0, 0, 0, 0]
  Logical : xbsIndex_r3/Logical  logical_function=AND  inputs=2  precision=Full  arith_type=Unsigned  n_bits=8  bin_pt=2  align_bp=on  latency=0  explicit_period=off  period=1  en=off  dbl_ovrd=off  show_param=off
      settings: xl_area=[0, 0, 0, 0, 0, 0, 0]
  Logical1 : xbsIndex_r3/Logical  logical_function=AND  inputs=3  precision=Full  arith_type=Unsigned  n_bits=8  bin_pt=2  align_bp=on  latency=0  explicit_period=on  period=1  en=off  dbl_ovrd=off  show_param=off
      settings: xl_area=[0, 0, 0, 0, 0, 0, 0]
  Logical2 : xbsIndex_r3/Logical  logical_function=AND  inputs=2  precision=Full  arith_type=Unsigned  n_bits=8  bin_pt=2  align_bp=on  latency=0  explicit_period=off  period=1  en=off  dbl_ovrd=off  show_param=off
      settings: xl_area=[0, 0, 0, 0, 0, 0, 0]
  Register1 : xbsIndex_r3/Register  init=0  reg_only_valid=off  explicit_period=on  period=1  rst=on  en=on  out_en=off  dbl_ovrd=off  show_param=off
      settings: xl_area=[0, 0, 0, 0, 0, 0, 0]
  Relational : xbsIndex_r3/Relational  mode=a=b  latency=1  explicit_period=off  period=1  en=off  dbl_ovrd=off  show_param=off
      settings: xl_area=[0, 0, 0, 0, 0, 0, 0]
  Relational1 : xbsIndex_r3/Relational  mode=a!=b  latency=1  explicit_period=on  period=1  en=on  dbl_ovrd=off  show_param=off
      settings: xl_area=[0, 0, 0, 0, 0, 0, 0]
  Scope7 : Scope  NumInputPorts=9
      settings: YMin=0~0~0~0~0~0.95~0~-5~-5  YMax=1~1100~7500~1~1~1.05~1~5~5  SaveName=ScopeData29
  last_read_tag : xbsIndex_r3/Register  init=0  reg_only_valid=off  explicit_period=off  period=1  rst=off  en=on  out_en=off  dbl_ovrd=off  show_param=off
      settings: xl_area=[0, 0, 0, 0, 0, 0, 0]
  negedge : Subsystem
  done : Outport
  wires:
  Logical2/1 -> Gateway Out1/1, Register1/2
  Gateway Out2/1 -> Scope7/9
  Gateway Out1/1 -> Scope7/8
  Gateway Out35/1 -> Scope7/7
  Gateway Out34/1 -> Scope7/6
  Gateway Out38/1 -> Scope7/4
  Gateway Out37/1 -> Scope7/5
  Gateway Out36/1 -> Scope7/3
  Gateway Out32/1 -> Scope7/2
  Gateway Out33/1 -> Scope7/1
  Convert/1 -> Register1/1, Register1/3
  Register1/1 -> Gateway Out35/1, done/1
  negedge/1(out) -> Gateway Out34/1, Convert/1
  Relational1/1 -> Logical2/1
  Counter/1 -> Gateway Out37/1, negedge/1(in)
  Logical1/1 -> Gateway Out38/1, Counter/1
  Relational/1 -> Gateway Out36/1, Logical1/1
  Delay1/1 -> Logical1/2
  rd_ack/1 -> Delay1/1
  Delay2/1 -> Logical1/3
  rd_valid/1 -> Delay2/1
  dram_data_tag/1 -> Relational/2
  last_read_tag/1 -> Gateway Out32/1, Relational1/2, Relational/1
  Logical/1 -> Logical2/2, Relational1/3, Gateway Out2/1, last_read_tag/2
  tag_in/1 -> Gateway Out33/1, Relational1/1, last_read_tag/1
  RWn/1 -> Logical/2
  cmd_valid/1 -> Logical/1

== system b_2x_8a_r309a/fmt_for_dram1/mk_4x32bit ==
  din : Inport  Port=1  LatchInput=off
  Concat3 : xbsIndex_r3/Concat  num_inputs=4  explicit_period=off  period=1  dbl_ovrd=off
  Convert{1..4} (4 alike) : xbsIndex_r3/Convert  arith_type="Signed  (2's comp)"  n_bits=32  bin_pt=0  quantization=Truncate  overflow=Wrap  latency=0  explicit_period=off  period=1  dbl_ovrd=off  show_param=off  inserted_by_tool=off  pipeline=off
      settings: xl_area=[0, 0, 0, 0, 0, 0, 0]
  Gateway Out{1..4,13..16} (8 alike) : xbsIndex_r3/Gateway Out  output_type=Double  nbits=8  bin_pt=6  arith_type=Boolean  quantization=Truncate  overflow=Wrap  hdl_port=off  timing_constraint=None  locs_specified=off  LOCs={}  needs_fixed_name=off  show_param=off
      settings: xl_area=[0, 0, 0, 0, 0, 0, 0]
  Reinterpret{,2,4,6} (4 alike) : xbsIndex_r3/Reinterpret  force_arith_type=on  arith_type=Unsigned  force_bin_pt=on  bin_pt=0  force_valid=on
  Reinterpret{1,3,5,7} (4 alike) : xbsIndex_r3/Reinterpret  force_arith_type=on  arith_type="Signed  (2's comp)"  force_bin_pt=on  bin_pt=0  force_valid=on
  Scope2 : Scope  NumInputPorts=8
      settings: YMin=0~0~0~0~0~0~0~0  YMax=20~20~20~20~20~20~20~20  SaveName=ScopeData3
  Slice10 : xbsIndex_r3/Slice  mode=Lower Bit Location + Width  nbits=(2*x_n_bits+1+x_int_bits)  bit1=0  base1=MSB of Input  bit0=2*(2*x_n_bits+1+x_int_bits)  base0=LSB of Input  boolean_output=off  explicit_period=off  period=1  dbl_ovrd=off
  Slice11 : xbsIndex_r3/Slice  mode=Lower Bit Location + Width  nbits=(2*x_n_bits+1+x_int_bits)  bit1=0  base1=MSB of Input  bit0=0  base0=LSB of Input  boolean_output=off  explicit_period=off  period=1  dbl_ovrd=off
  Slice12 : xbsIndex_r3/Slice  mode=Lower Bit Location + Width  nbits=(2*x_n_bits+1+x_int_bits)  bit1=0  base1=MSB of Input  bit0=(2*x_n_bits+1+x_int_bits)  base0=LSB of Input  boolean_output=off  explicit_period=off  period=1  dbl_ovrd=off
  Slice7 : xbsIndex_r3/Slice  mode=Lower Bit Location + Width  nbits=(2*x_n_bits+1+x_int_bits)  bit1=0  base1=MSB of Input  bit0=3*(2*x_n_bits+1+x_int_bits)  base0=LSB of Input  boolean_output=off  explicit_period=off  period=1  dbl_ovrd=off
  dout : Outport
  wires:
  Concat3/1 -> dout/1
  din/1 -> Slice12/1, Slice11/1, Slice10/1, Slice7/1
  Reinterpret6/1 -> Concat3/4
  Reinterpret4/1 -> Concat3/3
  Reinterpret2/1 -> Concat3/2
  Convert4/1 -> Reinterpret6/1, Gateway Out1/1
  Reinterpret7/1 -> Convert4/1, Gateway Out4/1
  Slice11/1 -> Reinterpret7/1
  Convert3/1 -> Reinterpret4/1, Gateway Out3/1
  Reinterpret5/1 -> Convert3/1, Gateway Out2/1
  Slice12/1 -> Reinterpret5/1
  Convert2/1 -> Reinterpret2/1, Gateway Out13/1
  Reinterpret3/1 -> Convert2/1, Gateway Out16/1
  Slice10/1 -> Reinterpret3/1
  Reinterpret/1 -> Concat3/1
  Convert1/1 -> Reinterpret/1, Gateway Out15/1
  Reinterpret1/1 -> Convert1/1, Gateway Out14/1
  Slice7/1 -> Reinterpret1/1
  Gateway Out14/1 -> Scope2/1
  Gateway Out15/1 -> Scope2/2
  Gateway Out16/1 -> Scope2/3
  Gateway Out13/1 -> Scope2/4
  Gateway Out2/1 -> Scope2/5
  Gateway Out3/1 -> Scope2/6
  Gateway Out4/1 -> Scope2/7
  Gateway Out1/1 -> Scope2/8

== system b_2x_8a_r309a/fmt_for_dram2/mk_4x32bit ==
  din : Inport  Port=1  LatchInput=off
  Concat3 : xbsIndex_r3/Concat  num_inputs=4  explicit_period=off  period=1  dbl_ovrd=off
  Convert{1..4} (4 alike) : xbsIndex_r3/Convert  arith_type="Signed  (2's comp)"  n_bits=32  bin_pt=0  quantization=Truncate  overflow=Wrap  latency=0  explicit_period=off  period=1  dbl_ovrd=off  show_param=off  inserted_by_tool=off  pipeline=off
      settings: xl_area=[0, 0, 0, 0, 0, 0, 0]
  Gateway Out{1..4,13..16} (8 alike) : xbsIndex_r3/Gateway Out  output_type=Double  nbits=8  bin_pt=6  arith_type=Boolean  quantization=Truncate  overflow=Wrap  hdl_port=off  timing_constraint=None  locs_specified=off  LOCs={}  needs_fixed_name=off  show_param=off
      settings: xl_area=[0, 0, 0, 0, 0, 0, 0]
  Reinterpret{,2,4,6} (4 alike) : xbsIndex_r3/Reinterpret  force_arith_type=on  arith_type=Unsigned  force_bin_pt=on  bin_pt=0  force_valid=on
  Reinterpret{1,3,5,7} (4 alike) : xbsIndex_r3/Reinterpret  force_arith_type=on  arith_type="Signed  (2's comp)"  force_bin_pt=on  bin_pt=0  force_valid=on
  Scope2 : Scope  NumInputPorts=8
      settings: YMin=0~0~0~0~0~0~0~0  YMax=20~20~20~20~20~20~20~20  SaveName=ScopeData3
  Slice10 : xbsIndex_r3/Slice  mode=Lower Bit Location + Width  nbits=(2*x_n_bits+1+x_int_bits)  bit1=0  base1=MSB of Input  bit0=2*(2*x_n_bits+1+x_int_bits)  base0=LSB of Input  boolean_output=off  explicit_period=off  period=1  dbl_ovrd=off
  Slice11 : xbsIndex_r3/Slice  mode=Lower Bit Location + Width  nbits=(2*x_n_bits+1+x_int_bits)  bit1=0  base1=MSB of Input  bit0=0  base0=LSB of Input  boolean_output=off  explicit_period=off  period=1  dbl_ovrd=off
  Slice12 : xbsIndex_r3/Slice  mode=Lower Bit Location + Width  nbits=(2*x_n_bits+1+x_int_bits)  bit1=0  base1=MSB of Input  bit0=(2*x_n_bits+1+x_int_bits)  base0=LSB of Input  boolean_output=off  explicit_period=off  period=1  dbl_ovrd=off
  Slice7 : xbsIndex_r3/Slice  mode=Lower Bit Location + Width  nbits=(2*x_n_bits+1+x_int_bits)  bit1=0  base1=MSB of Input  bit0=3*(2*x_n_bits+1+x_int_bits)  base0=LSB of Input  boolean_output=off  explicit_period=off  period=1  dbl_ovrd=off
  dout : Outport
  wires:
  Concat3/1 -> dout/1
  din/1 -> Slice12/1, Slice11/1, Slice10/1, Slice7/1
  Reinterpret6/1 -> Concat3/4
  Reinterpret4/1 -> Concat3/3
  Reinterpret2/1 -> Concat3/2
  Convert4/1 -> Reinterpret6/1, Gateway Out1/1
  Reinterpret7/1 -> Convert4/1, Gateway Out4/1
  Slice11/1 -> Reinterpret7/1
  Convert3/1 -> Reinterpret4/1, Gateway Out3/1
  Reinterpret5/1 -> Convert3/1, Gateway Out2/1
  Slice12/1 -> Reinterpret5/1
  Convert2/1 -> Reinterpret2/1, Gateway Out13/1
  Reinterpret3/1 -> Convert2/1, Gateway Out16/1
  Slice10/1 -> Reinterpret3/1
  Reinterpret/1 -> Concat3/1
  Convert1/1 -> Reinterpret/1, Gateway Out15/1
  Reinterpret1/1 -> Convert1/1, Gateway Out14/1
  Slice7/1 -> Reinterpret1/1
  Gateway Out14/1 -> Scope2/1
  Gateway Out15/1 -> Scope2/2
  Gateway Out16/1 -> Scope2/3
  Gateway Out13/1 -> Scope2/4
  Gateway Out2/1 -> Scope2/5
  Gateway Out3/1 -> Scope2/6
  Gateway Out4/1 -> Scope2/7
  Gateway Out1/1 -> Scope2/8

== system b_2x_8a_r309a/loopback/fwft_fifo ==
  din : Inport  Port=1  LatchInput=off
  we : Inport  Port=2  LatchInput=off
  ack : Inport  Port=3  LatchInput=off
  Convert : xbsIndex_r3/Convert  Orientation=left  arith_type=Boolean  n_bits=1  bin_pt=0  quantization=Truncate  overflow=Wrap  latency=0  explicit_period=off  period=1  dbl_ovrd=off  show_param=off  inserted_by_tool=off  pipeline=off
      settings: xl_area=[0, 0, 0, 0, 0, 0, 0]
  FIFO : xbsIndex_r3/FIFO  depth=256  percent_nbits=1  store_only_valid=on  init_zero=on  explicit_period=off  period=1  rst=off  en=off  use_almost_empty=off  almost_empty_offset=6  use_almost_full=off  almost_full_offset=6  dbl_ovrd=off  show_param=off  mem_type=Block RAM  gen_core=off
      settings: xl_area=[0, 0, 0, 0, 0, 0, 0]
  Inverter1 : xbsIndex_r3/Inverter  latency=0  explicit_period=off  period=1  en=off  dbl_ovrd=off  show_param=off
      settings: xl_area=[0, 0, 0, 0, 0, 0, 0]
  Logical1 : xbsIndex_r3/Logical  logical_function=OR  inputs=2  precision=Full  arith_type=Unsigned  n_bits=8  bin_pt=2  align_bp=on  latency=0  explicit_period=off  period=1  en=off  dbl_ovrd=off  show_param=off
      settings: xl_area=[0, 0, 0, 0, 0, 0, 0]
  Register2 : xbsIndex_r3/Register  init=0  reg_only_valid=off  explicit_period=on  period=1  rst=off  en=on  out_en=off  dbl_ovrd=off  show_param=off
      settings: xl_area=[0, 0, 0, 0, 0, 0, 0]
  dout : Outport
  valid : Outport  Port=2
  wires:
  din/1 -> FIFO/1
  we/1 -> FIFO/2
  FIFO/1 -> dout/1
  FIFO/2 -> Register2/1
  Logical1/1 -> FIFO/3, Register2/2
  ack/1 -> Logical1/1
  Register2/1 -> Convert/1, Inverter1/1
  Convert/1 -> Logical1/2
  Inverter1/1 -> valid/1
